simulink model "Feedback_dyn_outLoop"  (R2020b)
settings: Solver=FixedStepAuto  StartTime=0.0  StopTime=300  FixedStep=1e-3  RelTol=1e-3
values from neighbouring files (symbols this model uses):
  g_par = 9.81    [init.m]
  J_par = (M_par*4*l_par^2)/12    (= 192666666.667)    [init.m]
  l_par = 34    [init.m]
  M_par = 5e5    (= 500000)    [init.m]
  mu_x_par = 0.5*rho_par*cdx_par*Ax_par    (= 152.439)    [init.m]
  mu_y_par = 0.5*rho_par*cdy_par*Ay_par    (= 1.28880775561)    [init.m]
  T0 = M_par*g_par    (= 4905000)    [init.m]
  theta0 = deg2rad(15)    [init.m]
  x0 = 2    [init.m]
  y0 = -5    [init.m]
settings Model: Creator=chiara-s  LastModifiedBy=giorg

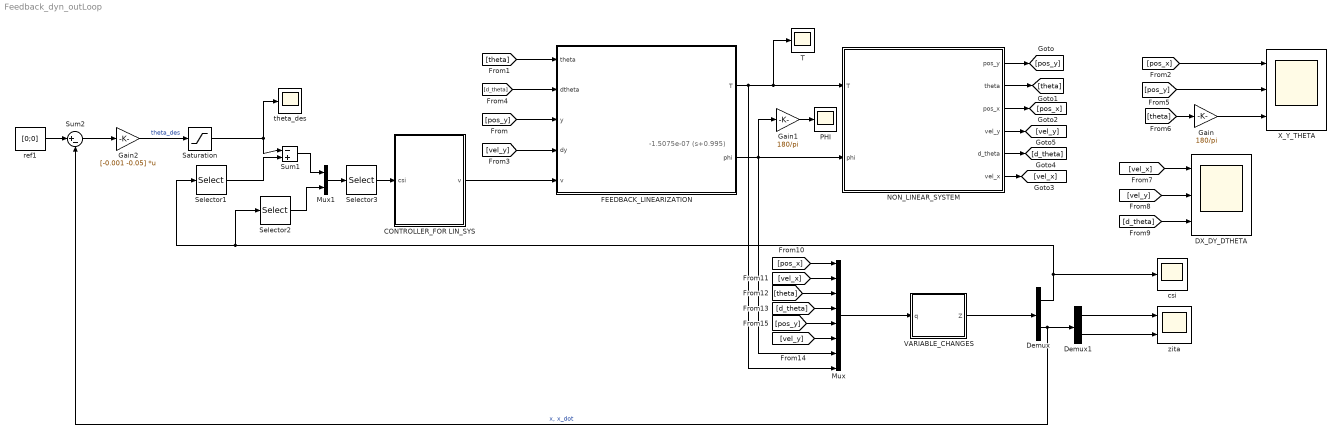
== system Feedback_dyn_outLoop ==
  note: -1.5075e-07 (s+0.995)
  CONTROLLER_FOR LIN_SYS : MATLAB Function  TreatAsAtomicUnit=on
  DX_DY_DTHETA : Scope  NumInputPorts=3
  Demux : Demux  Outputs=[6 2]
  Demux1 : Demux  Outputs=2
  FEEDBACK_LINEARIZATION : Subsystem
  Gain : Gain  Gain=180/pi
  Gain1 : Gain  Gain=180/pi
  Gain2 : Gain  Gain=[-0.001 -0.05]  Multiplication=Matrix(K*u)
  Mux : Mux  Inputs=8
  Mux1 : Mux  Inputs=2
  NON_LINEAR_SYSTEM : Subsystem
  PHI : Scope
  Saturation : Saturate  UpperLimit=0.2  LowerLimit=-0.2
  Selector1 : Selector  InputPortWidth=6  IndexOptions=Index vector (dialog)  Indices=[4]  OutputSizes=1
  Selector2 : Selector  InputPortWidth=6  IndexOptions=Index vector (dialog)  Indices=[1 2 3 5 6]  OutputSizes=1
  Selector3 : Selector  InputPortWidth=6  IndexOptions=Index vector (dialog)  Indices=[2 3 4 1 5 6]  OutputSizes=1
  Sum1 : Sum  Inputs=|-+
  Sum2 : Sum  Inputs=|+-
  T : Scope
  VARIABLE_CHANGES : MATLAB Function  TreatAsAtomicUnit=on
  X_Y_THETA : Scope  NumInputPorts=3
  csi : Scope
  ref1 : Constant  Value=[0;0]
  theta_des : Scope
  zita : Scope  NumInputPorts=2
  wires:
  NON_LINEAR_SYSTEM/1(pos_y) -> [pos_y]
  NON_LINEAR_SYSTEM/2(theta) -> [theta]
  NON_LINEAR_SYSTEM/3(pos_x) -> [pos_x]
  NON_LINEAR_SYSTEM/4(vel_y) -> [vel_y]
  NON_LINEAR_SYSTEM/5(d_theta) -> [d_theta]
  NON_LINEAR_SYSTEM/6(vel_x) -> [vel_x]
  [theta] -> FEEDBACK_LINEARIZATION/1(theta)
  [d_theta] -> FEEDBACK_LINEARIZATION/2(dtheta)
  [pos_y] -> FEEDBACK_LINEARIZATION/3(y)
  [vel_y] -> FEEDBACK_LINEARIZATION/4(dy)
  FEEDBACK_LINEARIZATION/1(T) -> NON_LINEAR_SYSTEM/1(T), T/1, Mux/8
  FEEDBACK_LINEARIZATION/2(phi) -> Mux/7, NON_LINEAR_SYSTEM/2(phi), Gain1/1
  CONTROLLER_FOR LIN_SYS/1(v) -> FEEDBACK_LINEARIZATION/5(v)
  [pos_x] -> Mux/1
  [vel_x] -> Mux/2
  [theta] -> Mux/3
  [d_theta] -> Mux/4
  [vel_y] -> Mux/6
  [pos_y] -> Mux/5
  Mux/1 -> VARIABLE_CHANGES/1(q)
  VARIABLE_CHANGES/1(Z) -> Demux/1
  Demux/1 -> csi/1, Selector2/1, Selector1/1
  [pos_x] -> X_Y_THETA/1
  [pos_y] -> X_Y_THETA/2
  [theta] -> Gain/1
  Gain/1 -> X_Y_THETA/3
  [vel_x] -> DX_DY_DTHETA/1
  [vel_y] -> DX_DY_DTHETA/2
  [d_theta] -> DX_DY_DTHETA/3
  Gain1/1 -> PHI/1
  Demux/2 -> Demux1/1, Sum2/2  "x, x_dot"
  Demux1/1 -> zita/1
  Demux1/2 -> zita/2
  Gain2/1 -> Saturation/1  "theta_des"
  Selector1/1 -> Sum1/2
  Sum1/1 -> Mux1/1
  Selector2/1 -> Mux1/2
  Mux1/1 -> Selector3/1
  Selector3/1 -> CONTROLLER_FOR LIN_SYS/1(csi)
  ref1/1 -> Sum2/1
  Sum2/1 -> Gain2/1
  Saturation/1 -> theta_des/1, Sum1/1

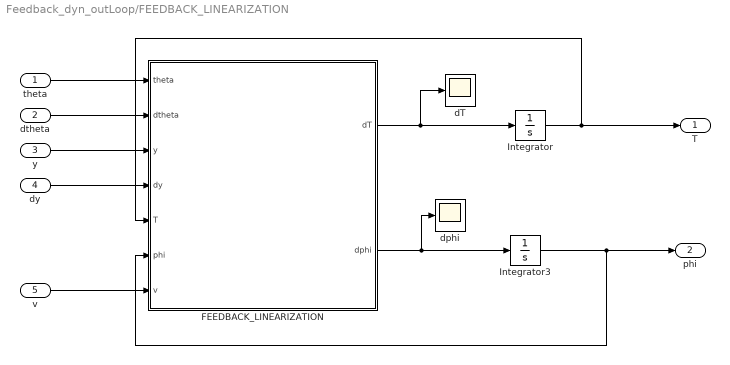
== system Feedback_dyn_outLoop/FEEDBACK_LINEARIZATION ==
  theta : Inport
  dtheta : Inport  Port=2
  y : Inport  Port=3
  dy : Inport  Port=4
  v : Inport  Port=5
  FEEDBACK_LINEARIZATION : MATLAB Function  TreatAsAtomicUnit=on
  Integrator : Integrator  InitialCondition=T0
  Integrator3 : Integrator
  dT : Scope
  dphi : Scope
  T : Outport
  phi : Outport  Port=2
  wires:
  FEEDBACK_LINEARIZATION/1(dT) -> dT/1, Integrator/1
  dy/1 -> FEEDBACK_LINEARIZATION/4(dy)
  theta/1 -> FEEDBACK_LINEARIZATION/1(theta)
  y/1 -> FEEDBACK_LINEARIZATION/3(y)
  Integrator/1 -> FEEDBACK_LINEARIZATION/5(T), T/1
  FEEDBACK_LINEARIZATION/2(dphi) -> dphi/1, Integrator3/1
  Integrator3/1 -> phi/1, FEEDBACK_LINEARIZATION/6(phi)
  dtheta/1 -> FEEDBACK_LINEARIZATION/2(dtheta)
  v/1 -> FEEDBACK_LINEARIZATION/7(v)

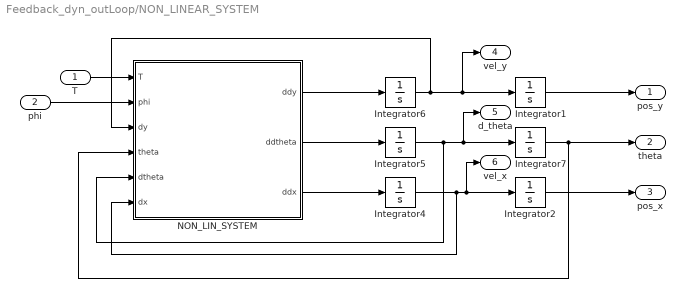
== system Feedback_dyn_outLoop/NON_LINEAR_SYSTEM ==
  T : Inport
  phi : Inport  Port=2
  Integrator1 : Integrator  InitialCondition=y0
  Integrator2 : Integrator  InitialCondition=x0
  Integrator4 : Integrator
  Integrator5 : Integrator
  Integrator6 : Integrator
  Integrator7 : Integrator  InitialCondition=theta0
  NON_LIN_SYSTEM : MATLAB Function  TreatAsAtomicUnit=on
  pos_y : Outport
  theta : Outport  Port=2
  pos_x : Outport  Port=3
  vel_y : Outport  Port=4
  d_theta : Outport  Port=5
  vel_x : Outport  Port=6
  wires:
  Integrator2/1 -> pos_x/1
  Integrator7/1 -> NON_LIN_SYSTEM/4(theta), theta/1
  NON_LIN_SYSTEM/2(ddtheta) -> Integrator5/1
  phi/1 -> NON_LIN_SYSTEM/2(phi)
  Integrator1/1 -> pos_y/1
  T/1 -> NON_LIN_SYSTEM/1(T)
  Integrator6/1 -> Integrator1/1, vel_y/1, NON_LIN_SYSTEM/3(dy)
  Integrator4/1 -> NON_LIN_SYSTEM/6(dx), vel_x/1, Integrator2/1
  NON_LIN_SYSTEM/1(ddy) -> Integrator6/1
  Integrator5/1 -> NON_LIN_SYSTEM/5(dtheta), Integrator7/1, d_theta/1
  NON_LIN_SYSTEM/3(ddx) -> Integrator4/1

== matlab function Feedback_dyn_outLoop/FEEDBACK_LINEARIZATION/FEEDBACK_LINEARIZATION ==
  data: dT output; dphi output; theta input; dtheta input; y input; dy input; T input; phi input; v input; M_par parameter; l_par parameter; J_par parameter; mu_y_par parameter; g_par parameter
function [dT, dphi] = fcn( theta, dtheta, y, dy, T, phi, v, M_par, l_par, J_par, mu_y_par, g_par)

E = zeros(2,2);
Gamma = zeros(2,1);

E =[cos(phi + theta)/M_par, -(T*sin(phi + theta))/M_par;
    -(l_par*sin(phi))/J_par,       -(T*l_par*cos(phi))/J_par];
 
Gamma = [(mu_y_par*((M_par*g_par + dy*mu_y_par)/M_par - (T*cos(phi + theta))/M_par))/M_par - (T*dtheta*sin(phi + theta))/M_par;
          0];

% v 2x1
u = -inv(E)*Gamma + inv(E)*v;
dT = u(1);
dphi = u(2);

end

== matlab function Feedback_dyn_outLoop/NON_LINEAR_SYSTEM/NON_LIN_SYSTEM ==
  data: T input; ddy output; phi input; dy input; theta input; dtheta input; dx input; ddtheta output; ddx output; M_par parameter; mu_x_par parameter; J_par parameter; l_par parameter; mu_y_par parameter; g_par parameter
function [ddy, ddtheta, ddx] = fcn(T, phi, dy, theta, dtheta, dx, M_par, mu_x_par, J_par, l_par, mu_y_par, g_par)

ddx = M_par^-1*(-T*sin(theta+phi) - mu_x_par*dx);
ddtheta = J_par^-1*(-T*l_par*sin(phi));
ddy = M_par^-1*(T*cos(theta+phi) - mu_y_par*dy - M_par*g_par);


end

== matlab function Feedback_dyn_outLoop/CONTROLLER_FOR LIN_SYS ==
  data: csi input; v output
function v = fcn(csi)

% v = K*csi;
%eigenvalues in [-1;-2;-3] for both subsystems (A1,B1) and (A2,B2)

% csi = [ csi(1) = y;
%         csi(2) = dy;
%         csi(3) = v1;
%         csi(4) = theta;
%         csi(5) = dtheta;
%         csi(6) = v2];

K = [-6 -11 -6   0   0  0;
      0   0  0  -6 -11 -6];
  
v = K*csi;

end

== matlab function Feedback_dyn_outLoop/VARIABLE_CHANGES ==
  data: q input; Z output; M_par parameter; g_par parameter; mu_y_par parameter; l_par parameter; J_par parameter
function Z = fcn(q, M_par, g_par, mu_y_par, l_par, J_par)

% q = [x dx theta dtheta y dy phi T];

Z = [ q(5); 
      q(6); 
      (q(8)*cos(q(7) + q(3)))/M_par - (M_par*g_par + q(6)*mu_y_par)/M_par;
      q(3);
      q(4);
      -(q(8)*l_par*sin(q(7)))/J_par;
      q(1);
      q(2)];

end
